simulink model "SpaceCraftAttitudeModel2"  (R2020b)
settings: Solver=VariableStepAuto  StartTime=0.0  StopTime=50  RelTol=1e-6
values from neighbouring files (symbols this model uses):
  Hwheel = [0;0;0.5]    [SimulinkSpacecraft.m]
  I = [1,0,0;0,4,0;0,0,0.5]    [SimulinkSpacecraft.m]
  invI = inv(I)    [SimulinkSpacecraft.m]
  Next = [0;0;0.0]    [SimulinkSpacecraft.m]
  Nthr = NMag    [SimulinkSpacecraft.m]
  omega1 = [0.05;0;0.05]    [SimulinkSpacecraft.m]
  stepTime = [5, 5+41.66]    [SimulinkSpacecraft.m]
libraries: vrlib x1
settings Model: Creator=Niels  LastModifiedBy=Niels

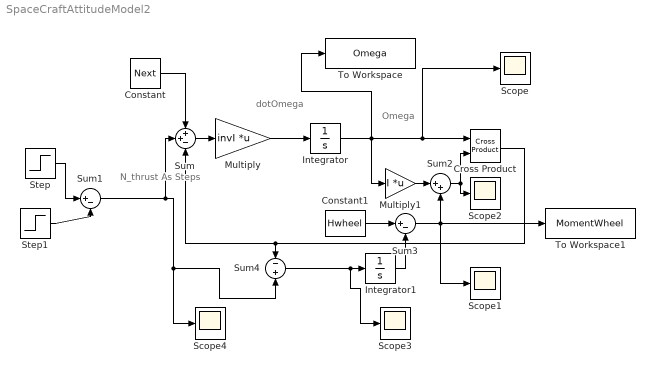
== system SpaceCraftAttitudeModel2 ==
  note: N_thrust
      | As Steps
  note: dotOmega
  note: Omega
  Constant : Constant  Value=Next
  Constant1 : Constant  Value=Hwheel
  Cross Product : vrlib/Utilities/Cross Product
  Integrator : Integrator  InitialCondition=omega1
  Integrator1 : Integrator
  Multiply : Gain  Gain=invI  Multiplication=Matrix(K*u)
  Multiply1 : Gain  Gain=I  Multiplication=Matrix(K*u)
  Scope{,1..4} (5 alike) : Scope
  Step : Step  Time=stepTime(1)  After=Nthr  SampleTime=0
  Step1 : Step  Time=stepTime(2)  After=Nthr  SampleTime=0
  Sum : Sum  Inputs=++-
  Sum1 : Sum  Inputs=|+-
  Sum2 : Sum  Inputs=|++
  Sum3 : Sum  Inputs=|+-
  Sum4 : Sum  Inputs=-+
  To Workspace : ToWorkspace  VariableName=Omega  SampleTime=-1
  To Workspace1 : ToWorkspace  VariableName=MomentWheel  SampleTime=-1
      settings: Save2DSignal=2-D array (concatenate along first dimension)
  wires:
  Multiply/1 -> Integrator/1
  Cross Product/1 -> Sum/3, Sum4/1
  Sum/1 -> Multiply/1
  Constant/1 -> Sum/1
  Integrator/1 -> Scope/1, Cross Product/1, To Workspace/1, Multiply1/1
  Sum1/1 -> Sum/2, Sum4/2, Scope4/1
  Constant1/1 -> Sum3/1
  Multiply1/1 -> Sum2/1
  Sum2/1 -> Scope2/1, Cross Product/2
  Sum3/1 -> To Workspace1/1, Sum2/2, Scope1/1
  Step1/1 -> Sum1/2
  Sum4/1 -> Scope3/1, Integrator1/1
  Integrator1/1 -> Sum3/2
  Step/1 -> Sum1/1
